simulink model "MIT"  (R2018a)
settings: Solver=ode45  StartTime=0.0  StopTime=100  RelTol=1e-3  EnableMultiTasking=on
settings Model: Creator=Jinlin Hao  LastModifiedBy=edward
settings DataIOCC: LimitDataPoints=on  SaveFormat=Array
settings OptimizationCC: LifeSpan=inf
settings DebuggingCC: SolverPrmCheckMsg=warning  SFUnexpectedBacktrackingDiag=warning  SFNoUnconditionalDefaultTransitionDiag=warning  SFExecutionAtInitializationDiag=none
settings HardwareCC: ProdBitPerPointer=32  ProdBitPerSizeT=32  ProdBitPerPtrDiffT=32  ProdLargestAtomicFloat=None  ProdIntDivRoundTo=Undefined  ProdEndianess=Unspecified  ProdWordSize=32  ProdHWDeviceType=32-bit Generic
settings ModelReferenceCC: PropagateSignalLabelsOutOfModel=off
settings CodeAppCC: StateflowObjectComments=on
settings GRTTargetCC: TargetLangStandard=C89/C90 (ANSI)  GeneratePreprocessorConditionals=Disable all
settings ConfigComp: CovMetricSettings=dw  CovHtmlReporting=on  CovSaveCumulativeToWorkspaceVar=on  CovSaveSingleToWorkspaceVar=on  CovExternalEMLEnable=off  CovSFcnEnable=off

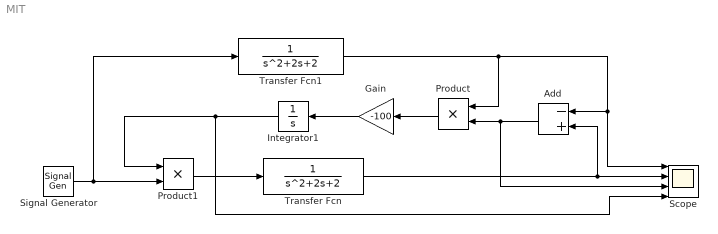
== system MIT ==
  Add : Sum  Inputs=-+
  Gain : Gain  Gain=-100
  Integrator1 : Integrator
  Product : Product
  Product1 : Product
  Scope : Scope  NumInputPorts=4
  Signal Generator : SignalGenerator  WaveForm=square  Frequency=0.1  Units=rad/sec
  Transfer Fcn : TransferFcn  Denominator=[1 2 2]
  Transfer Fcn1 : TransferFcn  Denominator=[1 2 2]
  wires:
  Product/1 -> Gain/1
  Gain/1 -> Integrator1/1
  Signal Generator/1 -> Transfer Fcn1/1, Product1/2
  Transfer Fcn1/1 -> Scope/1, Add/1, Product/1
  Product1/1 -> Transfer Fcn/1
  Transfer Fcn/1 -> Add/2, Scope/2
  Add/1 -> Scope/3, Product/2
  Integrator1/1 -> Scope/4, Product1/1
